simulink model "Closed_Loop_LQR"  (R2024a)
settings: Solver=FixedStepAuto  StartTime=0.0  StopTime=10  FixedStep=dt  RelTol=1e-3
values from neighbouring files (symbols this model uses):
  Amplitude_perturbation = 1    [A_a_Simulation_TrueSystem.m]    (also in B_a_Simulation_Model.m)
  B = full(B)    [A_b_TrueSystem.m]    (also in B_b_Model.m)
  bb = 1    [A_b_TrueSystem.m]    (also in B_b_Model.m)
  C_a = [zeros(N),eye(N)]    [A_b_TrueSystem.m]    (also in B_b_Model.m)
  C_q = [eye(N),zeros(N)]    [A_b_TrueSystem.m]    (also in B_b_Model.m)
  Constant_flow = 1    [A_a_Simulation_TrueSystem.m]    (also in B_a_Simulation_Model.m)
  Ctrue = zeros(2,2*N)    [A_b_TrueSystem.m]    (also in B_b_Model.m)
  Ei = full(Ei)    [A_b_TrueSystem.m]    (also in B_b_Model.m)
  Frequency_perturbation = pi/2    (= 1.57079632679)    [A_a_Simulation_TrueSystem.m]    (also in B_a_Simulation_Model.m)
  g = 9.8    [A_b_TrueSystem.m]    (also in B_b_Model.m)
  J = full(J)    [A_b_TrueSystem.m]    (also in B_b_Model.m)
  L = 10    [A_b_TrueSystem.m]    (also in B_b_Model.m)
  Psi = full(Psi)    [A_b_TrueSystem.m]    (also in B_b_Model.m; ModelForControl3.mat = ; TrueModel80.mat = )
  rho = 1    [A_b_TrueSystem.m]    (also in B_b_Model.m)
  T = blkdiag(eye(N)/bb,eye(N)/rho)    [A_b_TrueSystem.m]    (also in B_b_Model.m)
  X0 = [q0;alpha0]    [A_b_TrueSystem.m]    (also in B_b_Model.m)
undefined symbols (not defined in the file or in its folder): A_construit, B_construit, C_construit, K2, K_app_real, Yeq
settings Model: Creator=jptoledozu  LastModifiedBy=johnse

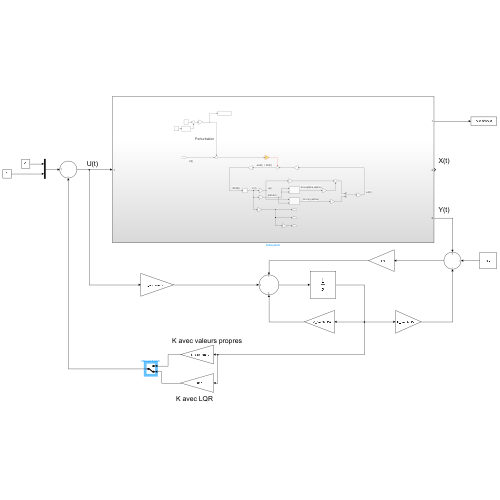
[thumbnail: Simulink's stored preview of the top-level diagram]
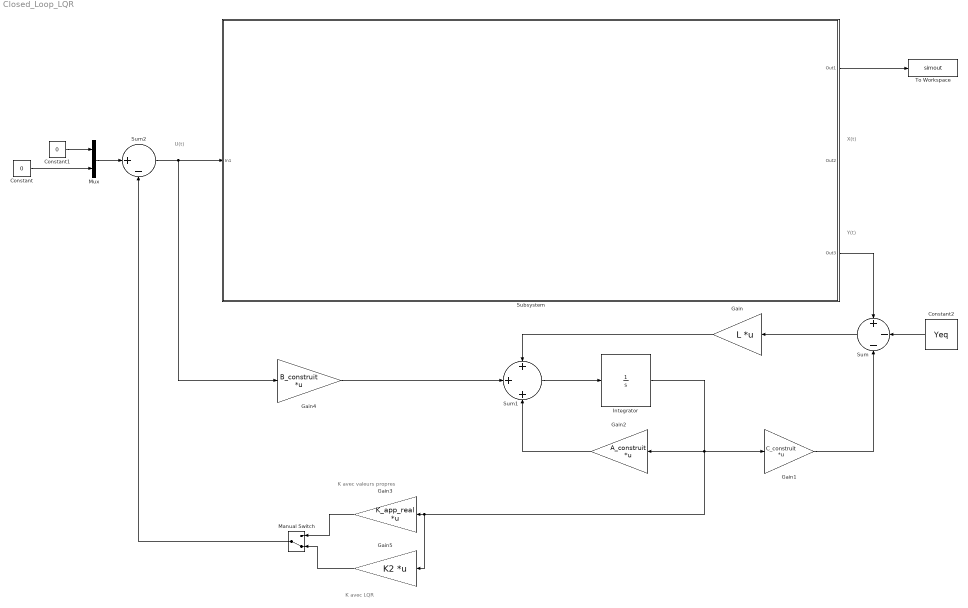
== system Closed_Loop_LQR ==
  note: Y(t)
  note: X(t)
  note: U(t)
  note: K avec valeurs propres
  note: K avec LQR
  Constant : Constant  Value=0
  Constant1 : Constant  Value=0
  Constant2 : Constant  Value=Yeq
  Gain : Gain  Gain=L  Multiplication=Matrix(K*u)
  Gain1 : Gain  Gain=C_construit  Multiplication=Matrix(K*u)
  Gain2 : Gain  Gain=A_construit  Multiplication=Matrix(K*u)
  Gain3 : Gain  Gain=K_app_real  Multiplication=Matrix(K*u)
  Gain4 : Gain  Gain=B_construit  Multiplication=Matrix(K*u)
  Gain5 : Gain  Gain=K2  Multiplication=Matrix(K*u)
  Integrator : Integrator
  Manual Switch : ManualSwitch  CurrentSetting=0
  Mux : Mux  Inputs=2
  Subsystem : Subsystem
  Sum : Sum  Inputs=+--
  Sum1 : Sum  Inputs=+++
  Sum2 : Sum  Inputs=|+-
  To Workspace : ToWorkspace  VariableName=simout  SaveFormat=Timeseries  SampleTime=-1
  wires:
  Subsystem/1(Out1) -> To Workspace/1
  Constant/1 -> Mux/2
  Constant1/1 -> Mux/1
  Subsystem/3(Out3) -> Sum/1
  Constant2/1 -> Sum/2
  Sum/1 -> Gain/1
  Gain/1 -> Sum1/1
  Sum1/1 -> Integrator/1
  Gain1/1 -> Sum/3
  Integrator/1 -> Gain5/1, Gain3/1, Gain1/1, Gain2/1
  Gain2/1 -> Sum1/3
  Mux/1 -> Sum2/1
  Sum2/1 -> Gain4/1, Subsystem/1(In1)
  Gain4/1 -> Sum1/2
  Gain3/1 -> Manual Switch/1
  Gain5/1 -> Manual Switch/2
  Manual Switch/1 -> Sum2/2

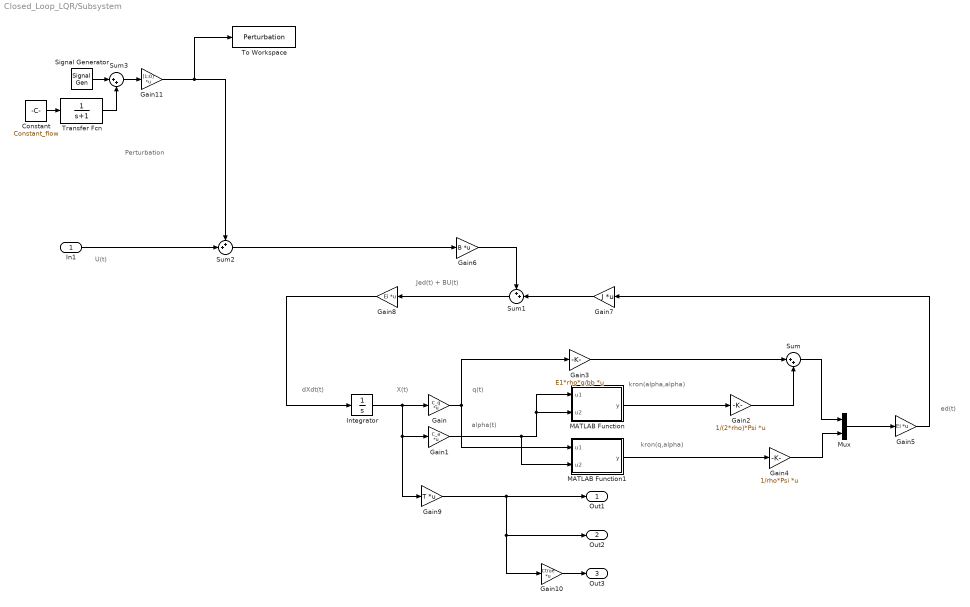
== system Closed_Loop_LQR/Subsystem ==
  note: Perturbation
  note: X(t)
  note: dXdt(t)
  note: q(t)
  note: alpha(t)
  note: kron(alpha,alpha)
  note: kron(q,alpha)
  note: ed(t)
  note: U(t)
  note: Jed(t) + BU(t)
  In1 : Inport
  Constant : Constant  Value=Constant_flow
  Gain : Gain  Gain=C_q  Multiplication=Matrix(K*u)
  Gain1 : Gain  Gain=C_a  Multiplication=Matrix(K*u)
  Gain10 : Gain  Gain=Ctrue  Multiplication=Matrix(K*u)
  Gain11 : Gain  Gain=[1;0]  Multiplication=Matrix(K*u)
  Gain2 : Gain  Gain=1/(2*rho)*Psi  Multiplication=Matrix(K*u)
  Gain3 : Gain  Gain=E1*rho*g/bb  Multiplication=Matrix(K*u)
  Gain4 : Gain  Gain=1/rho*Psi  Multiplication=Matrix(K*u)
  Gain5 : Gain  Gain=Ei  Multiplication=Matrix(K*u)
  Gain6 : Gain  Gain=B  Multiplication=Matrix(K*u)
  Gain7 : Gain  Gain=J  Multiplication=Matrix(K*u)
  Gain8 : Gain  Gain=Ei  Multiplication=Matrix(K*u)
  Gain9 : Gain  Gain=T  Multiplication=Matrix(K*u)
  Integrator : Integrator  InitialCondition=X0
  MATLAB Function : MATLAB Function  TreatAsAtomicUnit=on
  MATLAB Function1 : MATLAB Function  TreatAsAtomicUnit=on
  Mux : Mux  Inputs=2
  Signal Generator : SignalGenerator  Amplitude=Amplitude_perturbation  Frequency=Frequency_perturbation  Units=rad/sec
  Sum : Sum  Inputs=|++
  Sum1 : Sum  Inputs=++|
  Sum2 : Sum  Inputs=++|
  Sum3 : Sum  Inputs=|++
  To Workspace : ToWorkspace  VariableName=Perturbation  SaveFormat=Timeseries  SampleTime=-1
  Transfer Fcn : TransferFcn  Denominator=[1 1]
  Out1 : Outport
  Out2 : Outport  Port=2
  Out3 : Outport  Port=3
  wires:
  Gain5/1 -> Gain7/1
  MATLAB Function/1(y) -> Gain2/1
  Sum/1 -> Mux/1
  Mux/1 -> Gain5/1
  Gain/1 -> Gain3/1, MATLAB Function1/1(u1)
  Sum1/1 -> Gain8/1
  Gain2/1 -> Sum/2
  Gain7/1 -> Sum1/2
  Gain1/1 -> MATLAB Function1/2(u2), MATLAB Function/2(u2), MATLAB Function/1(u1)
  Gain4/1 -> Mux/2
  Integrator/1 -> Gain1/1, Gain9/1, Gain/1
  MATLAB Function1/1(y) -> Gain4/1
  Gain3/1 -> Sum/1
  In1/1 -> Sum2/2
  Gain9/1 -> Gain10/1, Out2/1, Out1/1
  Gain8/1 -> Integrator/1
  Gain6/1 -> Sum1/1
  Gain10/1 -> Out3/1
  Signal Generator/1 -> Sum3/1
  Sum2/1 -> Gain6/1
  Gain11/1 -> To Workspace/1, Sum2/1
  Constant/1 -> Transfer Fcn/1
  Sum3/1 -> Gain11/1
  Transfer Fcn/1 -> Sum3/2

== matlab function Closed_Loop_LQR/Subsystem/MATLAB Function ==
  data: u1 input; y output; u2 input
function y = fcn(u1,u2)

y = kron(u1,u2);

== matlab function Closed_Loop_LQR/Subsystem/MATLAB Function1 ==
  data: u1 input; y output; u2 input
function y = fcn(u1,u2)

y = kron(u1,u2);
